simulink model "Optical_Movement_Detection"  (Simulink 7.5)
settings: Solver=ode45  StartTime=0.0  StopTime=inf  RelTol=1e-3
values from neighbouring files (symbols this model uses):
  D = 1    [Copter_Animation.m]
  HSE_Bottom_1 = imresize(imread('D:\GoogleMapsBilder\PAR\HSE_Bottom_1.jpg'), 1)    [TESTS_Optical_Flow_Scenarios.m]
undefined symbols (not defined in the file or in its folder): dfilt, fspecial, imresize, Kanade, Low, Lucas, Rec, SDTV
libraries: simulink x17, dspobslib x12, vipgeotforms x5, dspsigops x4, dspmtrx3 x3, vipanalysis x3, dspstat3 x3, vipconversions x2, dspswit3 x2, vipsrcs x2, dsparch4 x1, dspsrcs4 x1
(part 2 of 2)

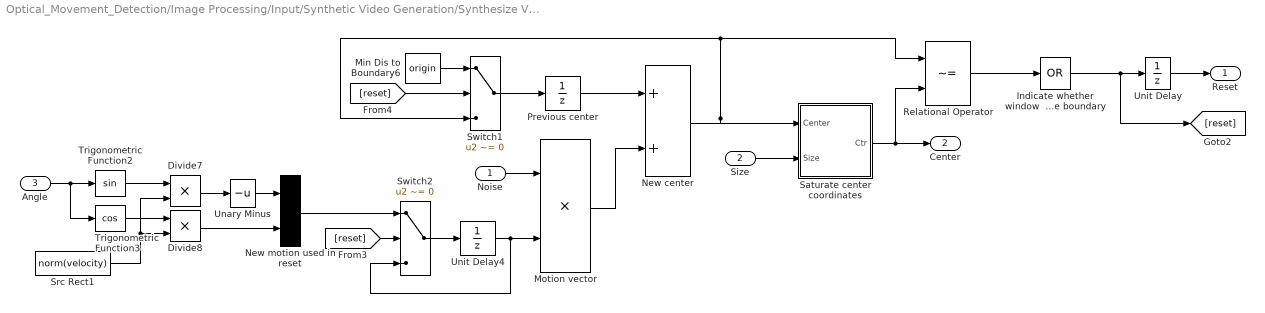
== system Optical_Movement_Detection/Image Processing/Input/Synthetic Video Generation/Synthesize Video/Center Locations ==
  Noise : Inport
  Size : Inport  Port=2  OutDataType=sfix(16)  OutScaling=2^0
  Angle : Inport  Port=3
  Divide7 : Product  Inputs=**  OutDataType=sfix(16)  OutScaling=2^-10
  Divide8 : Product  Inputs=**  OutDataType=sfix(16)  OutScaling=2^-10
  Indicate whether window  hit image boundary : Logic  Operator=OR  Inputs=1  AllPortsSameDT=off  OutDataTypeMode=boolean  OutDataTypeStr=boolean
  Min Dis to Boundary6 : Constant  Value=origin  OutDataType=sfix(16)  OutScaling=2^0
  Motion vector : Product  Inputs=**  OutDataType=sfix(16)  OutScaling=2^-10
  New center : Sum  OutDataType=sfix(16)  OutScaling=2^-10
  New motion used in reset : Concatenate  Mode=Vector
  Previous center : UnitDelay  X0=origin  SampleTime=-1
  Relational Operator : RelationalOperator  Operator=~=  LogicOutDataTypeMode=boolean  OutDataTypeStr=boolean
  Saturate center coordinates : Subsystem
  Src Rect1 : Constant  Value=norm(velocity)  VectorParams1D=off  OutDataType=sfix(16)  OutScaling=2^0  OutDataTypeStr=Inherit: Inherit via back propagation
  Switch1 : Switch  Criteria=u2 ~= 0  OutDataType=sfix(16)  OutScaling=2^0
  Switch2 : Switch  Criteria=u2 ~= 0  OutDataType=sfix(16)  OutScaling=2^0
  Trigonometric Function2 : Trigonometry
  Trigonometric Function3 : Trigonometry  Operator=cos
  Unary Minus : UnaryMinus
  Unit Delay : UnitDelay  X0=1  SampleTime=-1
  Unit Delay4 : UnitDelay  X0=velocity  SampleTime=-1
  Reset : Outport
  Center : Outport  Port=2
  wires:
  Unit Delay4/1 -> Switch2/3, Motion vector/2
  Previous center/1 -> New center/1
  [reset] -> Switch1/2
  [reset] -> Switch2/2
  Divide7/1 -> Unary Minus/1
  Unary Minus/1 -> New motion used in reset/1
  Divide8/1 -> New motion used in reset/2
  Src Rect1/1 -> Divide8/2, Divide7/2
  Switch1/1 -> Previous center/1
  Min Dis to Boundary6/1 -> Switch1/1
  Switch2/1 -> Unit Delay4/1
  New motion used in reset/1 -> Switch2/1
  Trigonometric Function3/1 -> Divide8/1
  Trigonometric Function2/1 -> Divide7/1
  Angle/1 -> Trigonometric Function3/1, Trigonometric Function2/1
  Relational Operator/1 -> Indicate whether window  hit image boundary/1
  Indicate whether window  hit image boundary/1 -> [reset], Unit Delay/1
  Saturate center coordinates/1(Ctr) -> Center/1, Relational Operator/2
  Size/1 -> Saturate center coordinates/2(Size)
  New center/1 -> Switch1/3, Relational Operator/1, Saturate center coordinates/1(Center)
  Unit Delay/1 -> Reset/1
  Motion vector/1 -> New center/2
  Noise/1 -> Motion vector/1

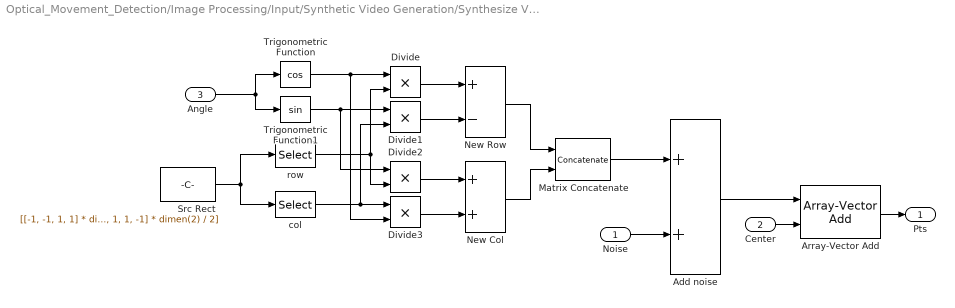
== system Optical_Movement_Detection/Image Processing/Input/Synthetic Video Generation/Synthesize Video/Corner Locations ==
  Noise : Inport
  Center : Inport  Port=2
  Angle : Inport  Port=3
  Add noise : Sum  OutDataType=sfix(16)  OutScaling=2^-10
  Array-Vector Add : dspmtrx3/Array-Vector Add  DialogController=dspDDGCreate  DialogControllerArgs=DataTag6  Dimension=1  V_Source=Input port  V_VectFromMask=[0.5 0.25]  firstCoeffDataTypeStr=Inherit: Same word length as input  firstCoeffLastDataTypeStr=Inherit: Same word length as input  firstCoeffMin=[]  firstCoeffMax=[]  outputDataTypeStr=Inherit: Same as accumulator  outputLastDataTypeStr=Inherit: Same as accumulator  outputMin=[]  outputMax=[]  roundingMode=Floor  overflowMode=off
  Divide{,1..3} (4 alike) : Product  Inputs=**  OutDataType=sfix(16)  OutScaling=2^-10
  Matrix Concatenate : Concatenate  Mode=Multidimensional array
  New Col : Sum  OutDataType=sfix(16)  OutScaling=2^-10
  New Row : Sum  Inputs=+-  OutDataType=sfix(16)  OutScaling=2^-10
  Src Rect : Constant  Value=[[-1, -1, 1, 1] * dimen(1) / 2; [-1, 1, 1, -1] * dimen(2) / 2]  OutDataType=sfix(16)  OutScaling=2^0
  Trigonometric Function : Trigonometry  Operator=cos
  Trigonometric Function1 : Trigonometry
  col : Selector  NumberOfDimensions=2  IndexMode=Zero-based  InputPortWidth=3  IndexOptions=Index vector (dialog),Select all  Indices=1,1  OutputSizes=1,1
  row : Selector  NumberOfDimensions=2  IndexMode=Zero-based  InputPortWidth=3  IndexOptions=Index vector (dialog),Select all  Indices=0,1  OutputSizes=1,1
  Pts : Outport
  wires:
  Noise/1 -> Add noise/2
  Center/1 -> Array-Vector Add/2
  Array-Vector Add/1 -> Pts/1
  Src Rect/1 -> col/1, row/1
  Divide2/1 -> New Col/1
  Divide3/1 -> New Col/2
  New Row/1 -> Matrix Concatenate/1
  New Col/1 -> Matrix Concatenate/2
  Matrix Concatenate/1 -> Add noise/1
  Angle/1 -> Trigonometric Function/1, Trigonometric Function1/1
  Divide/1 -> New Row/1
  Divide1/1 -> New Row/2
  Trigonometric Function/1 -> Divide3/2, Divide/1
  Trigonometric Function1/1 -> Divide2/1, Divide1/1
  row/1 -> Divide2/2, Divide/2
  col/1 -> Divide1/2, Divide3/1
  Add noise/1 -> Array-Vector Add/1

== system Optical_Movement_Detection/Image Processing/Optical Flow/Corner Features OF/Corner Matching/Calculate Distances ==
  F1 : Inport  OutDataType=sfix(16)  OutScaling=2^0
  N1 : Inport  Port=2  OutDataType=sfix(16)  OutScaling=2^0
  F2 : Inport  Port=3  OutDataType=sfix(16)  OutScaling=2^0
  N2 : Inport  Port=4  OutDataType=sfix(16)  OutScaling=2^0
  For Iterator Subsystem : Subsystem  TreatAsAtomicUnit=on
  Initial Values1 : Constant  Value=maxNum  OutDataType=sfix(16)  OutScaling=2^0  OutDataTypeStr=Inherit: Inherit via back propagation  SampleTime=-1
  Initial Values2 : Constant  Value=maxNum  OutDataType=sfix(16)  OutScaling=2^0  OutDataTypeStr=Inherit: Inherit via back propagation  SampleTime=-1
  MinMax1 : MinMax  Inputs=2  OutDataType=sfix(16)  OutScaling=2^0
  MinMax2 : MinMax  Inputs=2  OutDataType=sfix(16)  OutScaling=2^0
  Dis : Outport  OutDataType=sfix(16)  OutScaling=2^0
  wires:
  MinMax2/1 -> For Iterator Subsystem/4(N2)
  F2/1 -> For Iterator Subsystem/3(F2)
  MinMax1/1 -> For Iterator Subsystem/2(N1)
  F1/1 -> For Iterator Subsystem/1(F1)
  For Iterator Subsystem/1(Dis) -> Dis/1
  N2/1 -> MinMax2/2
  Initial Values2/1 -> MinMax2/1
  N1/1 -> MinMax1/2
  Initial Values1/1 -> MinMax1/1

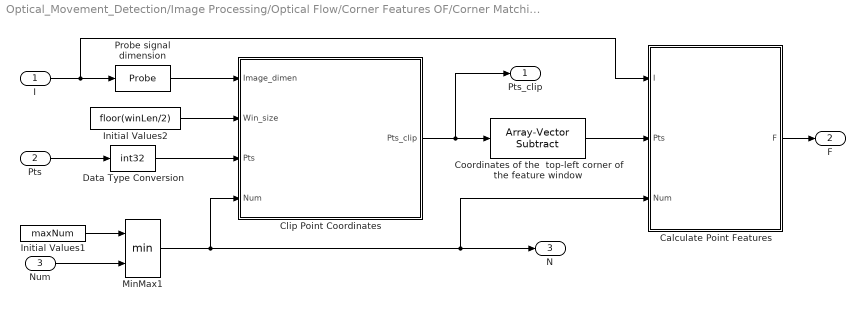
== system Optical_Movement_Detection/Image Processing/Optical Flow/Corner Features OF/Corner Matching/Calculate Features ==
  I : Inport  OutDataType=sfix(16)  OutScaling=2^0
  Pts : Inport  Port=2  OutDataType=sfix(16)  OutScaling=2^0
  Num : Inport  Port=3  OutDataType=sfix(16)  OutScaling=2^0
  Calculate Point Features : Subsystem
  Clip Point Coordinates : Subsystem
  Coordinates of the  top-left corner of the feature window : dspmtrx3/Array-Vector Subtract  DialogController=dspDDGCreate  DialogControllerArgs=DataTag10  Dimension=1  V_Source=Dialog parameter  V_VectFromMask=floor([winLen; winLen] / 2)  firstCoeffDataTypeStr=Inherit: Same word length as input  firstCoeffLastDataTypeStr=Inherit: Same word length as input  firstCoeffMin=[]  firstCoeffMax=[]  outputMin=[]  outputMax=[]  roundingMode=Floor  overflowMode=off
  Data Type Conversion : DataTypeConversion  OutDataTypeMode=int32  OutDataType=sfix(16)  OutScaling=2^0  OutDataTypeStr=int32
  Initial Values1 : Constant  Value=maxNum  OutDataType=sfix(16)  OutScaling=2^0  OutDataTypeStr=Inherit: Inherit via back propagation  SampleTime=-1
  Initial Values2 : Constant  Value=floor(winLen/2)  OutDataType=sfix(16)  OutScaling=2^0  OutDataTypeStr=Inherit: Inherit via back propagation  SampleTime=-1
  MinMax1 : MinMax  Inputs=2  OutDataType=sfix(16)  OutScaling=2^0
  Probe signal dimension : Probe  ProbeWidth=off  ProbeSampleTime=off  ProbeComplexSignal=off  ProbeSignalDimensions=on  ProbeDimensionsDataType=int32
  Pts_clip : Outport  OutDataType=sfix(16)  OutScaling=2^0
  F : Outport  Port=2  OutDataType=sfix(16)  OutScaling=2^0
  N : Outport  Port=3  OutDataType=sfix(16)  OutScaling=2^0
  wires:
  Data Type Conversion/1 -> Clip Point Coordinates/3(Pts)
  MinMax1/1 -> N/1, Calculate Point Features/3(Num), Clip Point Coordinates/4(Num)
  Coordinates of the  top-left corner of the feature window/1 -> Calculate Point Features/2(Pts)
  Clip Point Coordinates/1(Pts_clip) -> Coordinates of the  top-left corner of the feature window/1, Pts_clip/1
  Pts/1 -> Data Type Conversion/1
  Initial Values2/1 -> Clip Point Coordinates/2(Win_size)
  Probe signal dimension/1 -> Clip Point Coordinates/1(Image_dimen)
  I/1 -> Calculate Point Features/1(I), Probe signal dimension/1
  Initial Values1/1 -> MinMax1/1
  Num/1 -> MinMax1/2
  Calculate Point Features/1(F) -> F/1

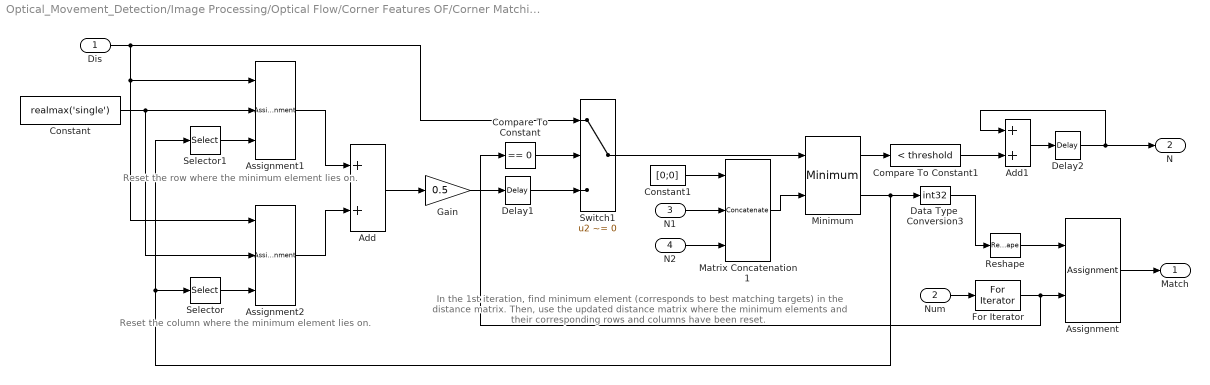
== system Optical_Movement_Detection/Image Processing/Optical Flow/Corner Features OF/Corner Matching/Find Best Matches ==
  note: In the 1st iteration, find minimum element (corresponds to
      | best matching targets) in the distance matrix. Then, use the
      | updated distance matrix where the minimum elements and
      | their  corresponding rows and columns have been reset.
  note: Reset the column where the
      | minimum element lies on.
  note: Reset the row where the
      | minimum element lies on.
  Dis : Inport  OutDataType=sfix(16)  OutScaling=2^0
  Num : Inport  Port=2  OutDataType=sfix(16)  OutScaling=2^0
  N1 : Inport  Port=3  OutDataType=sfix(16)  OutScaling=2^0
  N2 : Inport  Port=4  OutDataType=sfix(16)  OutScaling=2^0
  Add : Sum  OutDataType=sfix(16)  OutScaling=2^-10
  Add1 : Sum  OutDataTypeMode=int32  OutDataType=sfix(16)  OutScaling=2^-10  OutDataTypeStr=int32
  Assignment : Assignment  NumberOfDimensions=2  IndexMode=Zero-based  OutputInitialize=Specify size for each dimension in table  IndexOptions=Assign all,Index vector (port)  Indices=-1,-1  OutputSizes=2,maxNum
  Assignment1 : Assignment  NumberOfDimensions=2  IndexMode=Zero-based  IndexOptions=Index vector (port),Assign all  Indices=1,-1  OutputSizes=1,1
  Assignment2 : Assignment  NumberOfDimensions=2  IndexMode=Zero-based  IndexOptions=Assign all,Index vector (port)  Indices=-1,-1  OutputSizes=1,1
  Compare To Constant : simulink/Logic and Bit Operations/Compare To Constant  SystemSampleTime=-1  relop===  const=0  LogicOutDataTypeMode=boolean  ZeroCross=off
  Compare To Constant1 : simulink/Logic and Bit Operations/Compare To Constant  SystemSampleTime=-1  relop=<  const=threshold  LogicOutDataTypeMode=uint8  ZeroCross=off
  Constant : Constant  Value=realmax('single')  VectorParams1D=off  OutDataType=sfix(16)  OutScaling=2^0  OutDataTypeStr=Inherit: Inherit via back propagation
  Constant1 : Constant  Value=[0;0]  VectorParams1D=off  OutDataType=sfix(16)  OutScaling=2^0  OutDataTypeStr=Inherit: Inherit via back propagation
  Data Type  Conversion3 : DataTypeConversion  OutDataTypeMode=int32  OutDataType=sfix(16)  OutScaling=2^0  OutDataTypeStr=int32  SaturateOnIntegerOverflow=on  RndMeth=Zero
  Delay1 : dspsigops/Delay  dly_unit=Samples  delay=1  ic_detail=off  dif_ic_for_ch=off  dif_ic_for_dly=off  ic=0  reset_popup=None
  Delay2 : dspsigops/Delay  dly_unit=Samples  delay=1  ic_detail=off  dif_ic_for_ch=off  dif_ic_for_dly=off  ic=0  reset_popup=None
  For Iterator : ForIterator  ResetStates=reset  IterationSource=external  IterationLimit=expLaneNum  IndexMode=Zero-based
  Gain : Gain  Gain=0.5  ParameterDataType=sfix(16)  ParameterScaling=2^0  OutDataType=sfix(16)  OutScaling=2^0
  Matrix Concatenation1 : Concatenate  NumInputs=3  Mode=Multidimensional array
  Minimum : dspstat3/Minimum  DialogController=dspDDGCreate  DialogControllerArgs=DataTag11  fcn=Value and Index  reset=None  indexBase=Zero  operateOver=Entire input  Dimension=1  colComp=on  operation=minimum  roiEnable=on  roiType=Rectangles  roiPortion=Entire ROI  roiOutput=Individual statistics for each ROI  roiFlag=off  roundingMode=Floor  overflowMode=off
  Reshape : Reshape  OutputDimensionality=Column vector (2-D)
  Selector : Selector  IndexMode=Zero-based  InputPortWidth=2  IndexOptions=Index vector (dialog)  Indices=1  OutputSizes=1
  Selector1 : Selector  IndexMode=Zero-based  InputPortWidth=2  IndexOptions=Index vector (dialog)  Indices=0  OutputSizes=1
  Switch1 : Switch  Criteria=u2 ~= 0  OutDataType=sfix(16)  OutScaling=2^0
  Match : Outport  OutDataType=sfix(16)  OutScaling=2^0
  N : Outport  Port=2  OutDataType=sfix(16)  OutScaling=2^0
  wires:
  Gain/1 -> Delay1/1
  Minimum/1 -> Compare To Constant1/1
  Compare To Constant1/1 -> Add1/2
  Delay2/1 -> Add1/1, N/1
  Add1/1 -> Delay2/1
  Num/1 -> For Iterator/1
  Data Type  Conversion3/1 -> Reshape/1
  Compare To Constant/1 -> Switch1/2
  For Iterator/1 -> Compare To Constant/1, Assignment/2
  Switch1/1 -> Minimum/1
  Dis/1 -> Switch1/1, Assignment2/1, Assignment1/1
  Delay1/1 -> Switch1/3
  Assignment/1 -> Match/1
  Selector1/1 -> Assignment1/3
  Assignment1/1 -> Add/1
  Assignment2/1 -> Add/2
  Add/1 -> Gain/1
  Minimum/2 -> Data Type  Conversion3/1, Selector/1, Selector1/1
  Constant/1 -> Assignment1/2, Assignment2/2
  Selector/1 -> Assignment2/3
  Constant1/1 -> Matrix Concatenation1/1
  N1/1 -> Matrix Concatenation1/2
  N2/1 -> Matrix Concatenation1/3
  Matrix Concatenation1/1 -> Minimum/2
  Reshape/1 -> Assignment/1

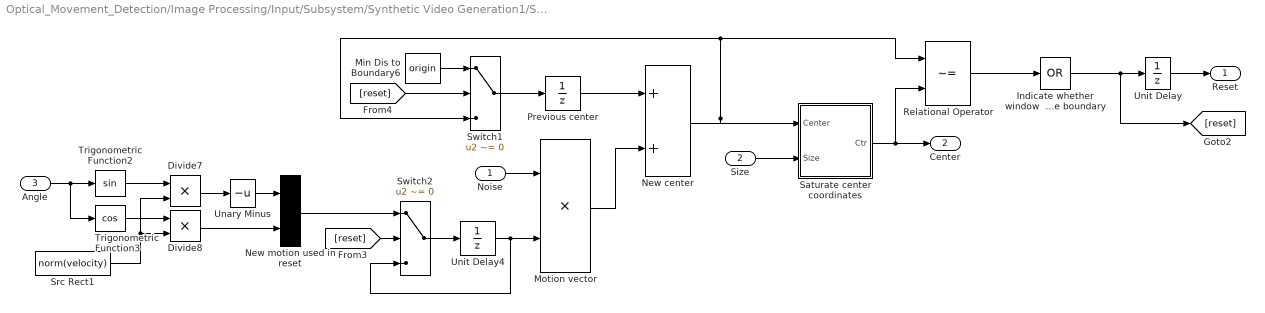
== system Optical_Movement_Detection/Image Processing/Input/Subsystem/Synthetic Video Generation1/Synthesize Video/Center Locations ==
  Noise : Inport
  Size : Inport  Port=2  OutDataType=sfix(16)  OutScaling=2^0
  Angle : Inport  Port=3
  Divide7 : Product  Inputs=**  OutDataType=sfix(16)  OutScaling=2^-10
  Divide8 : Product  Inputs=**  OutDataType=sfix(16)  OutScaling=2^-10
  Indicate whether window  hit image boundary : Logic  Operator=OR  Inputs=1  AllPortsSameDT=off  OutDataTypeMode=boolean  OutDataTypeStr=boolean
  Min Dis to Boundary6 : Constant  Value=origin  OutDataType=sfix(16)  OutScaling=2^0
  Motion vector : Product  Inputs=**  OutDataType=sfix(16)  OutScaling=2^-10
  New center : Sum  OutDataType=sfix(16)  OutScaling=2^-10
  New motion used in reset : Concatenate  Mode=Vector
  Previous center : UnitDelay  X0=origin  SampleTime=-1
  Relational Operator : RelationalOperator  Operator=~=  LogicOutDataTypeMode=boolean  OutDataTypeStr=boolean
  Saturate center coordinates : Subsystem
  Src Rect1 : Constant  Value=norm(velocity)  VectorParams1D=off  OutDataType=sfix(16)  OutScaling=2^0  OutDataTypeStr=Inherit: Inherit via back propagation
  Switch1 : Switch  Criteria=u2 ~= 0  OutDataType=sfix(16)  OutScaling=2^0
  Switch2 : Switch  Criteria=u2 ~= 0  OutDataType=sfix(16)  OutScaling=2^0
  Trigonometric Function2 : Trigonometry
  Trigonometric Function3 : Trigonometry  Operator=cos
  Unary Minus : UnaryMinus
  Unit Delay : UnitDelay  X0=1  SampleTime=-1
  Unit Delay4 : UnitDelay  X0=velocity  SampleTime=-1
  Reset : Outport
  Center : Outport  Port=2
  wires:
  Unit Delay4/1 -> Switch2/3, Motion vector/2
  Previous center/1 -> New center/1
  [reset] -> Switch1/2
  [reset] -> Switch2/2
  Divide7/1 -> Unary Minus/1
  Unary Minus/1 -> New motion used in reset/1
  Divide8/1 -> New motion used in reset/2
  Src Rect1/1 -> Divide8/2, Divide7/2
  Switch1/1 -> Previous center/1
  Min Dis to Boundary6/1 -> Switch1/1
  Switch2/1 -> Unit Delay4/1
  New motion used in reset/1 -> Switch2/1
  Trigonometric Function3/1 -> Divide8/1
  Trigonometric Function2/1 -> Divide7/1
  Angle/1 -> Trigonometric Function3/1, Trigonometric Function2/1
  Relational Operator/1 -> Indicate whether window  hit image boundary/1
  Indicate whether window  hit image boundary/1 -> [reset], Unit Delay/1
  Saturate center coordinates/1(Ctr) -> Center/1, Relational Operator/2
  Size/1 -> Saturate center coordinates/2(Size)
  New center/1 -> Switch1/3, Relational Operator/1, Saturate center coordinates/1(Center)
  Unit Delay/1 -> Reset/1
  Motion vector/1 -> New center/2
  Noise/1 -> Motion vector/1

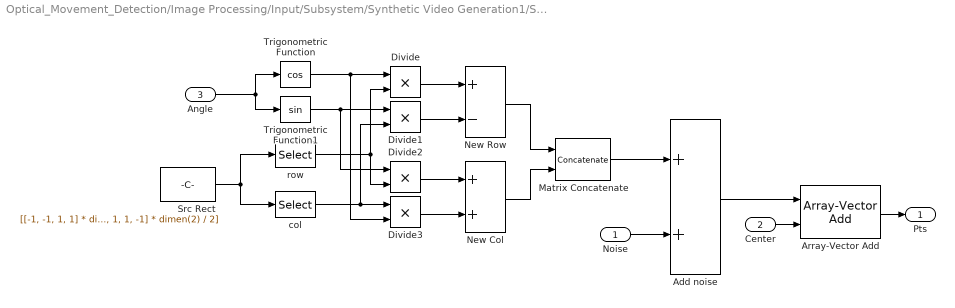
== system Optical_Movement_Detection/Image Processing/Input/Subsystem/Synthetic Video Generation1/Synthesize Video/Corner Locations ==
  Noise : Inport
  Center : Inport  Port=2
  Angle : Inport  Port=3
  Add noise : Sum  OutDataType=sfix(16)  OutScaling=2^-10
  Array-Vector Add : dspmtrx3/Array-Vector Add  DialogController=dspDDGCreate  DialogControllerArgs=DataTag2  Dimension=1  V_Source=Input port  V_VectFromMask=[0.5 0.25]  firstCoeffDataTypeStr=Inherit: Same word length as input  firstCoeffLastDataTypeStr=Inherit: Same word length as input  firstCoeffMin=[]  firstCoeffMax=[]  outputDataTypeStr=Inherit: Same as accumulator  outputLastDataTypeStr=Inherit: Same as accumulator  outputMin=[]  outputMax=[]  roundingMode=Floor  overflowMode=off
  Divide{,1..3} (4 alike) : Product  Inputs=**  OutDataType=sfix(16)  OutScaling=2^-10
  Matrix Concatenate : Concatenate  Mode=Multidimensional array
  New Col : Sum  OutDataType=sfix(16)  OutScaling=2^-10
  New Row : Sum  Inputs=+-  OutDataType=sfix(16)  OutScaling=2^-10
  Src Rect : Constant  Value=[[-1, -1, 1, 1] * dimen(1) / 2; [-1, 1, 1, -1] * dimen(2) / 2]  OutDataType=sfix(16)  OutScaling=2^0
  Trigonometric Function : Trigonometry  Operator=cos
  Trigonometric Function1 : Trigonometry
  col : Selector  NumberOfDimensions=2  IndexMode=Zero-based  InputPortWidth=3  IndexOptions=Index vector (dialog),Select all  Indices=1,1  OutputSizes=1,1
  row : Selector  NumberOfDimensions=2  IndexMode=Zero-based  InputPortWidth=3  IndexOptions=Index vector (dialog),Select all  Indices=0,1  OutputSizes=1,1
  Pts : Outport
  wires:
  Noise/1 -> Add noise/2
  Center/1 -> Array-Vector Add/2
  Array-Vector Add/1 -> Pts/1
  Src Rect/1 -> col/1, row/1
  Divide2/1 -> New Col/1
  Divide3/1 -> New Col/2
  New Row/1 -> Matrix Concatenate/1
  New Col/1 -> Matrix Concatenate/2
  Matrix Concatenate/1 -> Add noise/1
  Angle/1 -> Trigonometric Function/1, Trigonometric Function1/1
  Divide/1 -> New Row/1
  Divide1/1 -> New Row/2
  Trigonometric Function/1 -> Divide3/2, Divide/1
  Trigonometric Function1/1 -> Divide2/1, Divide1/1
  row/1 -> Divide2/2, Divide/2
  col/1 -> Divide1/2, Divide3/1
  Add noise/1 -> Array-Vector Add/1

== system Optical_Movement_Detection/Image Processing/Input/Synthetic Video Generation/Synthesize Video/Center Locations/Saturate center coordinates ==
  Center : Inport
  Size : Inport  Port=2
  Center2 : Sum  Inputs=-+  OutDataType=sfix(16)  OutScaling=2^-10
  Min Dis to Boundary : Constant  Value=kron([ceil(sqrt(dimen(1)^2+dimen(2)^2)/2)], [1; 1])  OutDataType=sfix(16)  OutScaling=2^0
  MinMax : MinMax  Function=max  Inputs=2  OutDataType=sfix(16)  OutScaling=2^0
  MinMax1 : MinMax  Inputs=2  OutDataType=sfix(16)  OutScaling=2^0
  row1 : Selector  IndexMode=Zero-based  InputPortWidth=3  IndexOptions=Index vector (dialog)  Indices=[0 1]  OutputSizes=1
  Ctr : Outport
  wires:
  Size/1 -> row1/1
  MinMax1/1 -> Ctr/1
  Center/1 -> MinMax/1
  Center2/1 -> MinMax1/2
  MinMax/1 -> MinMax1/1
  row1/1 -> Center2/2
  Min Dis to Boundary/1 -> Center2/1, MinMax/2

== system Optical_Movement_Detection/Image Processing/Optical Flow/Corner Features OF/Corner Matching/Calculate Distances/For Iterator Subsystem ==
  F1 : Inport  OutDataType=sfix(16)  OutScaling=2^0
  N1 : Inport  Port=2  OutDataType=sfix(16)  OutScaling=2^0
  F2 : Inport  Port=3  OutDataType=sfix(16)  OutScaling=2^0
  N2 : Inport  Port=4  OutDataType=sfix(16)  OutScaling=2^0
  For Iterator : ForIterator  IterationSource=external  IndexMode=Zero-based
  For Iterator Subsystem : Subsystem  TreatAsAtomicUnit=on
  Select feature  for 1 corner : Selector  NumberOfDimensions=2  IndexMode=Zero-based  InputPortWidth=2  IndexOptions=Select all,Index vector (port)  Indices=0,1  OutputSizes=1,1
  Update feature  for a corner : Assignment  NumberOfDimensions=2  IndexMode=Zero-based  OutputInitialize=Specify size for each dimension in table  IndexOptions=Assign all,Index vector (port)  Indices=1,1  OutputSizes=maxNum,maxNum
  Dis : Outport  OutDataType=sfix(16)  OutScaling=2^0
  wires:
  Update feature  for a corner/1 -> Dis/1
  N1/1 -> For Iterator Subsystem/2(N1)
  F1/1 -> For Iterator Subsystem/1(F1)
  Select feature  for 1 corner/1 -> For Iterator Subsystem/3(f2)
  F2/1 -> Select feature  for 1 corner/1
  For Iterator/1 -> Select feature  for 1 corner/2, Update feature  for a corner/2
  N2/1 -> For Iterator/1
  For Iterator Subsystem/1(Dis) -> Update feature  for a corner/1

== system Optical_Movement_Detection/Image Processing/Optical Flow/Corner Features OF/Corner Matching/Calculate Features/Calculate Point Features ==
  note: Calculate feature for a corner.
  I : Inport
  Pts : Inport  Port=2
  Num : Inport  Port=3
  For Iterator : ForIterator  IterationSource=external  IndexMode=Zero-based
  Reshape : Reshape  OutputDimensionality=Column vector (2-D)
  Selector : Selector  NumberOfDimensions=2  IndexMode=Zero-based  InputPortWidth=3  IndexOptions=Starting index (port),Starting index (port)  Indices=[1 3],1  OutputSizes=winLen,winLen
  Selector1 : Selector  NumberOfDimensions=2  IndexMode=Zero-based  InputPortWidth=3  IndexOptions=Select all,Index vector (port)  Indices=[1 3],1  OutputSizes=9,9
  Selector2 : Selector  IndexMode=Zero-based  InputPortWidth=2  IndexOptions=Index vector (dialog)  Indices=0  OutputSizes=9
  Selector3 : Selector  IndexMode=Zero-based  InputPortWidth=2  IndexOptions=Index vector (dialog)  Indices=1  OutputSizes=9
  Update Feature  for a Corner : Assignment  NumberOfDimensions=2  IndexMode=Zero-based  OutputInitialize=Specify size for each dimension in table  IndexOptions=Assign all,Index vector (port)  Indices=1,1  OutputSizes=winLen^2,maxNum
  F : Outport
  wires:
  Selector3/1 -> Selector/3
  Selector2/1 -> Selector/2
  Num/1 -> For Iterator/1
  Update Feature  for a Corner/1 -> F/1
  Pts/1 -> Selector1/1
  I/1 -> Selector/1
  Reshape/1 -> Update Feature  for a Corner/1
  Selector/1 -> Reshape/1
  Selector1/1 -> Selector2/1, Selector3/1
  For Iterator/1 -> Update Feature  for a Corner/2, Selector1/2

== system Optical_Movement_Detection/Image Processing/Optical Flow/Corner Features OF/Corner Matching/Calculate Features/Clip Point Coordinates ==
  Image_dimen : Inport  OutDataType=sfix(16)  OutScaling=2^0
  Win_size : Inport  Port=2  OutDataType=sfix(16)  OutScaling=2^0
  Pts : Inport  Port=3
  Num : Inport  Port=4
  Add : Sum  Inputs=-+  OutDataType=sfix(16)  OutScaling=2^-10
  Bias : Bias  Bias=-1
  Clip row/col coordinates : Subsystem
  For i = 0: 1 (select row/col) : ForIterator  IterationLimit=2  IndexMode=Zero-based
  Selector1 : Selector  NumberOfDimensions=2  IndexMode=Zero-based  InputPortWidth=3  IndexOptions=Index vector (port),Select all  Indices=[1 3],1  OutputSizes=9,9
  Selector2 : Selector  IndexMode=Zero-based  InputPortWidth=2  IndexOptions=Index vector (port)  Indices=[1 3]  OutputSizes=9
  Update Coordinates : Assignment  NumberOfDimensions=2  IndexMode=Zero-based  IndexOptions=Index vector (port),Assign all  Indices=1,1  OutputSizes=81,50
  Pts_clip : Outport  OutDataType=sfix(16)  OutScaling=2^0
  wires:
  Selector2/1 -> Add/2
  For i = 0: 1 (select row/col)/1 -> Selector1/2, Selector2/2, Update Coordinates/3
  Clip row/col coordinates/1(Coordinates_clip) -> Update Coordinates/2
  Bias/1 -> Clip row/col coordinates/2(High)
  Update Coordinates/1 -> Pts_clip/1
  Num/1 -> Clip row/col coordinates/4(Num)
  Selector1/1 -> Clip row/col coordinates/3(Coordinates)
  Win_size/1 -> Add/1, Clip row/col coordinates/1(Low)
  Add/1 -> Bias/1
  Image_dimen/1 -> Selector2/1
  Pts/1 -> Update Coordinates/1, Selector1/1

== system Optical_Movement_Detection/Image Processing/Input/Subsystem/Synthetic Video Generation1/Synthesize Video/Center Locations/Saturate center coordinates ==
  Center : Inport
  Size : Inport  Port=2
  Center2 : Sum  Inputs=-+  OutDataType=sfix(16)  OutScaling=2^-10
  Min Dis to Boundary : Constant  Value=kron([ceil(sqrt(dimen(1)^2+dimen(2)^2)/2)], [1; 1])  OutDataType=sfix(16)  OutScaling=2^0
  MinMax : MinMax  Function=max  Inputs=2  OutDataType=sfix(16)  OutScaling=2^0
  MinMax1 : MinMax  Inputs=2  OutDataType=sfix(16)  OutScaling=2^0
  row1 : Selector  IndexMode=Zero-based  InputPortWidth=3  IndexOptions=Index vector (dialog)  Indices=[0 1]  OutputSizes=1
  Ctr : Outport
  wires:
  Size/1 -> row1/1
  MinMax1/1 -> Ctr/1
  Center/1 -> MinMax/1
  Center2/1 -> MinMax1/2
  MinMax/1 -> MinMax1/1
  row1/1 -> Center2/2
  Min Dis to Boundary/1 -> Center2/1, MinMax/2

== system Optical_Movement_Detection/Image Processing/Optical Flow/Corner Features OF/Corner Matching/Calculate Distances/For Iterator Subsystem/For Iterator Subsystem ==
  F1 : Inport  OutDataType=sfix(16)  OutScaling=2^0
  N1 : Inport  Port=2  OutDataType=sfix(16)  OutScaling=2^0
  f2 : Inport  Port=3  OutDataType=sfix(16)  OutScaling=2^0
  Distance between two feature vectors : Subsystem
  For Iterator : ForIterator  IterationSource=external  IndexMode=Zero-based
  Select feature  for 1 corner : Selector  NumberOfDimensions=2  IndexMode=Zero-based  InputPortWidth=2  IndexOptions=Select all,Index vector (port)  Indices=0,1  OutputSizes=1,1
  Update feature  for a corner : Assignment  NumberOfDimensions=2  IndexMode=Zero-based  OutputInitialize=Specify size for each dimension in table  IndexOptions=Index vector (port),Assign all  Indices=1,1  OutputSizes=maxNum,1
  Dis : Outport  OutDataType=sfix(16)  OutScaling=2^0
  wires:
  Select feature  for 1 corner/1 -> Distance between two feature vectors/1(f1)
  f2/1 -> Distance between two feature vectors/2(f2)
  Update feature  for a corner/1 -> Dis/1
  F1/1 -> Select feature  for 1 corner/1
  For Iterator/1 -> Select feature  for 1 corner/2, Update feature  for a corner/2
  N1/1 -> For Iterator/1
  Distance between two feature vectors/1(dis) -> Update feature  for a corner/1

== system Optical_Movement_Detection/Image Processing/Optical Flow/Corner Features OF/Corner Matching/Calculate Features/Clip Point Coordinates/Clip row/col coordinates ==
  Low : Inport  OutDataType=sfix(16)  OutScaling=2^0
  High : Inport  Port=2  OutDataType=sfix(16)  OutScaling=2^0
  Coordinates : Inport  Port=3
  Num : Inport  Port=4  OutDataType=sfix(16)  OutScaling=2^0
  Clip a Coordinate : Subsystem
  For Iterator : ForIterator  IterationSource=external  IterationLimit=2  IndexMode=Zero-based
  Select Coordinate of a Point : Selector  NumberOfDimensions=2  IndexMode=Zero-based  InputPortWidth=3  IndexOptions=Select all,Index vector (port)  Indices=[1 3],1  OutputSizes=9,1
  Update Feature  for a Corner : Assignment  NumberOfDimensions=2  IndexMode=Zero-based  IndexOptions=Assign all,Index vector (port)  Indices=1,1  OutputSizes=81,50
  Coordinates_clip : Outport  OutDataType=sfix(16)  OutScaling=2^0
  wires:
  Clip a Coordinate/1(Coordinate_clip) -> Update Feature  for a Corner/2
  Update Feature  for a Corner/1 -> Coordinates_clip/1
  High/1 -> Clip a Coordinate/2(High)
  Low/1 -> Clip a Coordinate/1(Low)
  Select Coordinate of a Point/1 -> Clip a Coordinate/3(Coordinate)
  Num/1 -> For Iterator/1
  Coordinates/1 -> Update Feature  for a Corner/1, Select Coordinate of a Point/1
  For Iterator/1 -> Select Coordinate of a Point/2, Update Feature  for a Corner/3

== system Optical_Movement_Detection/Image Processing/Optical Flow/Corner Features OF/Corner Matching/Calculate Distances/For Iterator Subsystem/For Iterator Subsystem/Distance between two feature vectors ==
  f1 : Inport  OutDataType=sfix(16)  OutScaling=2^0
  f2 : Inport  Port=2  OutDataType=sfix(16)  OutScaling=2^0
  Abs : Abs  OutDataType=sfix(16)  OutScaling=2^0
  Add : Sum  Inputs=+-  OutDataType=sfix(16)  OutScaling=2^-10
  Sum of Elements : Sum  Inputs=+  OutDataType=sfix(16)  OutScaling=2^-10
  dis : Outport  OutDataType=sfix(16)  OutScaling=2^0
  wires:
  Sum of Elements/1 -> dis/1
  Abs/1 -> Sum of Elements/1
  Add/1 -> Abs/1
  f2/1 -> Add/2
  f1/1 -> Add/1

== system Optical_Movement_Detection/Image Processing/Optical Flow/Corner Features OF/Corner Matching/Calculate Features/Clip Point Coordinates/Clip row/col coordinates/Clip a Coordinate ==
  Low : Inport  OutDataType=sfix(16)  OutScaling=2^0
  High : Inport  Port=2  OutDataType=sfix(16)  OutScaling=2^0
  Coordinate : Inport  Port=3  OutDataType=sfix(16)  OutScaling=2^0
  MinMax1 : MinMax  Function=max  Inputs=2  OutDataType=sfix(16)  OutScaling=2^0
  MinMax2 : MinMax  Inputs=2  OutDataType=sfix(16)  OutScaling=2^0
  Coordinate_clip : Outport  OutDataType=sfix(16)  OutScaling=2^0
  wires:
  MinMax2/1 -> Coordinate_clip/1
  High/1 -> MinMax2/2
  MinMax1/1 -> MinMax2/1
  Low/1 -> MinMax1/2
  Coordinate/1 -> MinMax1/1

== matlab function Image Processing/Optical Flow/Optical Flow Segmentation in Sectors Corner Features/Optical Flow Lines1 ==
  data: vel_Values input double; Cam_Img_Dim input double; vel_Lines output double; Omega_avg output double; scaleFactor parameter double size=1
function [vel_Lines, Omega_avg]=OpticalFlowLines(vel_Values, Cam_Img_Dim,scaleFactor) 

% Generates the coordinate points of optical flow lines

persistent first_time;
persistent X;
persistent Y;
persistent RV;
persistent CV;

%persistent Max_Vec_Length;

persistent Origin_Re;
persistent Origin_Im;

persistent Sec_1_Cnt;
persistent Sec_2_Cnt;
persistent Sec_3_Cnt;
persistent Sec_4_Cnt;

persistent Sec_1;
persistent Sec_2;
persistent Sec_3;
persistent Sec_4;

persistent R;
persistent C;
persistent Test_mat;
persistent med_vel_val;

%med_vel_val=median(vel_Values);
%[R C] = size(med_vel_val);
if isempty(first_time)
    first_time     = 1;
    Origin_Re = Cam_Img_Dim(1)/2%double(176);
    [R C] = size(vel_Values)
    Origin_Im = Cam_Img_Dim(2)/2%double(144);
end

Sec_1 = double(0);
Sec_2 = double(0);
Sec_3 = double(0);
Sec_4 = double(0);

Sec_1_Cnt = 1;
Sec_2_Cnt = 1;
Sec_3_Cnt = 1;
Sec_4_Cnt = 1;

%sectors
%       ^Im
%       |         
%   4   |  1
%-------------->Re
%   3   |  2
%       |

% for i=1:R
%     for k=1:C
%       j=vel_Values(i,k);
%     if(real(j)>=0) % Sec_1 or Sec_2
%         if(imag(j)>=0) %Sec_1
%             Sec_1_Cnt=Sec_1_Cnt+1;
%             Sec_1=Sec_1+double(abs(j))
%         else           %Sec_2
%             Sec_2_Cnt=Sec_2_Cnt+1;
%             Sec_2=Sec_2+double(abs(j))
%         end
%     else            % Sec_3 or Sec_4
%         if(imag(j)>=0) %Sec_4
%             Sec_4_Cnt=Sec_4_Cnt+1;
%             Sec_4=Sec_4+double(abs(j))
%         else           %Sec_3
%             Sec_3_Cnt=Sec_3_Cnt+1;
%             Sec_3=Sec_3+double(abs(j))
%         end
%     end
%     end
% end

%Other segm
for i=1:R
    for k=1:C
      j=vel_Values(i,k);
    if(real(j)>=0) % Sec_1 or Sec_2
        Sec_1_Cnt=Sec_1_Cnt+1;
        Sec_1=Sec_1+double(abs(real(j)));
        if(imag(j)>=0) %Sec_2
            Sec_2_Cnt=Sec_2_Cnt+1;
            Sec_2=Sec_2+double(imag(j));
        else           %Sec_4
            Sec_4_Cnt=Sec_4_Cnt+1;
            Sec_4=Sec_4+double(imag(j));
        end
    else            % Sec_3 or Sec_4
        Sec_3_Cnt=Sec_3_Cnt+1;
        Sec_3=Sec_3+double(abs(real(j)));
        if(imag(j)>=0) %Sec_2
            Sec_2_Cnt=Sec_2_Cnt+1;
            Sec_2=Sec_2+double(imag(j));
        else           %Sec_4
            Sec_4_Cnt=Sec_4_Cnt+1;
            Sec_4=Sec_4+double(imag(j));
        end
    end
    end
end


% Sec_1_Mat = vel_Values((real(vel_Values) >= 0) & (imag(vel_Values) >= 0));
% Sec_2_Mat = vel_Values((real(vel_Values) >= 0) & (imag(vel_Values) < 0));
% Sec_3_Mat = vel_Values((real(vel_Values) < 0) & (imag(vel_Values) < 0));
% Sec_4_Mat = vel_Values((real(vel_Values) < 0) & (imag(vel_Values) >= 0));


% Sec_1 = sum(abs(Sec_1_Mat)/(size(Sec_1_Mat, 1)*size(Sec_1_Mat, 2)));
% Sec_2 = sum(abs(Sec_1_Mat)/(size(Sec_1_Mat, 1)*size(Sec_1_Mat, 2)));
% Sec_3 = sum(abs(Sec_1_Mat)/(size(Sec_1_Mat, 1)*size(Sec_1_Mat, 2)));
% Sec_4 = sum(abs(Sec_1_Mat)/(size(Sec_1_Mat, 1)*size(Sec_1_Mat, 2)));

Sec_1 = Sec_1/Sec_1_Cnt;
Sec_2 = Sec_2/Sec_2_Cnt;
Sec_3 = Sec_3/Sec_3_Cnt;
Sec_4 = Sec_4/Sec_4_Cnt;

% Omega_Re_Plus = (scaleFactor*(Sec_1+Sec_2))/2
% Omega_Re_Minus = (scaleFactor*(Sec_3+Sec_4))/2
% Omega_Im_Plus = (scaleFactor*(Sec_1+Sec_4))/2
% Omega_Im_Minus = (scaleFactor*(Sec_3+Sec_2))/2

Omega_Re_Plus = scaleFactor*Sec_1; %Sec_2
Omega_Re_Minus = scaleFactor*Sec_3; %Sec_4
Omega_Im_Plus = scaleFactor*Sec_4; %Sec_1
Omega_Im_Minus = scaleFactor*Sec_2; %Sec_3

%Calculation of rotation

rotation_comp=min([abs(Omega_Re_Plus) abs(Omega_Re_Minus) abs(Omega_Im_Plus) abs(Omega_Im_Minus)]);

if(rotation_comp>0)
    Omega_avg = [abs(Omega_Re_Plus)-rotation_comp abs(Omega_Re_Minus)-rotation_comp abs(Omega_Im_Plus)-rotation_comp abs(Omega_Im_Minus)-rotation_comp rotation_comp];
else
    Omega_avg = [abs(Omega_Re_Plus) abs(Omega_Re_Minus) abs(Omega_Im_Plus) abs(Omega_Im_Minus) rotation_comp];
end


vel_Lines = [[Origin_Im Origin_Im Origin_Im Origin_Im];[Origin_Re Origin_Re Origin_Re Origin_Re];...
[Origin_Im Origin_Im+abs(Omega_Im_Minus) Origin_Im Origin_Im-abs(Omega_Im_Plus)];[Origin_Re+abs(Omega_Re_Plus) Origin_Re Origin_Re-abs(Omega_Re_Minus) Origin_Re]];

== matlab function Image Processing/Optical Flow/Cross for callibration/Optical Flow Lines1 ==
  data: vel_Values input double; Cam_Img_Dim input double; vel_Lines output double
function vel_Lines =OpticalFlowLines(vel_Values, Cam_Img_Dim) 

% Generates the coordinate points of optical flow lines

persistent first_time;
persistent X;
persistent Y;
persistent RV;
persistent CV;

%persistent Max_Vec_Length;

persistent Origin_Re;
persistent Origin_Im;

persistent Sec_1_Cnt;
persistent Sec_2_Cnt;
persistent Sec_3_Cnt;
persistent Sec_4_Cnt;

persistent Sec_1;
persistent Sec_2;
persistent Sec_3;
persistent Sec_4;

persistent R;
persistent C;
persistent Test_mat;
persistent med_vel_val;

%med_vel_val=median(vel_Values);
%[R C] = size(med_vel_val);
if isempty(first_time)
    first_time     = 1;
    Origin_Re = Cam_Img_Dim(1)/2%double(176);
    [R C] = size(vel_Values)
    Origin_Im = Cam_Img_Dim(2)/2%double(144);
end


Omega_Re_Plus = 700;
Omega_Re_Minus = 700;
Omega_Im_Plus = 700;
Omega_Im_Minus = 700;


vel_Lines = [[Origin_Im Origin_Im Origin_Im Origin_Im];[Origin_Re Origin_Re Origin_Re Origin_Re];...
[Origin_Im Origin_Im+abs(Omega_Im_Minus) Origin_Im Origin_Im-abs(Omega_Im_Plus)];[Origin_Re+abs(Omega_Re_Plus) Origin_Re Origin_Re-abs(Omega_Re_Minus) Origin_Re]];

== matlab function Image Processing/Optical Flow/Corner Features OF/Embedded MATLAB Function ==
  data: vec output double; Tform input double; allowNewCalc input double; rot output double; TsOpt input double
function [vec, rot] = clc(Tform, allowNewCalc, TsOpt)
%#eml
persistent vec_old;
persistent rot_old;
persistent first_time;
persistent db_3_filter;

if isempty(first_time)
    vec_old = double(complex(0,0));
    vec = double(complex(0,0));
    rot = double(0);
    rot_old = double(0);
    first_time=1;
    db_3_filter=double([0;0;0;0;0;0;0]);
end
    Tform
    %v'=Tform*v with v=[x y 1]^T and v'=[x' y' 1]
    if(allowNewCalc)
    vec=double(complex(Tform(2,3),Tform(1,3)));
    rot=double(abs(-asin(complex(Tform(1,2)))))/TsOpt;
    %Detect direction of rotation
    if((Tform(1,3) > 0) && Tform(2,3) < 0)
        %counterclockwise is negative
        rot=rot*(-1);
    end
    db_3_filter=circshift(db_3_filter, 1);
    db_3_filter(1,1)=rot;
    db_3_filter
    rot=sum(db_3_filter)/7;
    vec_old=vec;
    rot_old=rot;
else
vec=vec_old;
rot=rot_old;
end

== matlab function Image Processing/Optical Flow/Optical Flow Segmentation in Sectors Block Matching/Optical Flow Lines1 ==
  data: vel_Values input double; Cam_Img_Dim input double; vel_Lines output double; Omega_avg output double; scaleFactor parameter double size=1
function [vel_Lines, Omega_avg]=OpticalFlowLines(vel_Values, Cam_Img_Dim,scaleFactor) 

% Generates the coordinate points of optical flow lines

persistent first_time;
persistent X;
persistent Y;
persistent RV;
persistent CV;

%persistent Max_Vec_Length;

persistent Origin_Re;
persistent Origin_Im;

persistent Sec_1_Cnt;
persistent Sec_2_Cnt;
persistent Sec_3_Cnt;
persistent Sec_4_Cnt;

persistent Sec_1;
persistent Sec_2;
persistent Sec_3;
persistent Sec_4;

persistent R;
persistent C;
persistent Test_mat;
persistent med_vel_val;

%med_vel_val=median(vel_Values);
%[R C] = size(med_vel_val);
if isempty(first_time)
    first_time     = 1;
    Origin_Re = Cam_Img_Dim(1)/2%double(176);
    [R C] = size(vel_Values)
    Origin_Im = Cam_Img_Dim(2)/2%double(144);
end

Sec_1 = double(0);
Sec_2 = double(0);
Sec_3 = double(0);
Sec_4 = double(0);

Sec_1_Cnt = 1;
Sec_2_Cnt = 1;
Sec_3_Cnt = 1;
Sec_4_Cnt = 1;

%sectors
%       ^Im
%       |         
%   4   |  1
%-------------->Re
%   3   |  2
%       |

% for i=1:R
%     for k=1:C
%       j=vel_Values(i,k);
%     if(real(j)>=0) % Sec_1 or Sec_2
%         if(imag(j)>=0) %Sec_1
%             Sec_1_Cnt=Sec_1_Cnt+1;
%             Sec_1=Sec_1+double(abs(j))
%         else           %Sec_2
%             Sec_2_Cnt=Sec_2_Cnt+1;
%             Sec_2=Sec_2+double(abs(j))
%         end
%     else            % Sec_3 or Sec_4
%         if(imag(j)>=0) %Sec_4
%             Sec_4_Cnt=Sec_4_Cnt+1;
%             Sec_4=Sec_4+double(abs(j))
%         else           %Sec_3
%             Sec_3_Cnt=Sec_3_Cnt+1;
%             Sec_3=Sec_3+double(abs(j))
%         end
%     end
%     end
% end

%Other segm
for i=1:R
    for k=1:C
      j=vel_Values(i,k);
    if(real(j)>=0) % Sec_1 or Sec_2
        Sec_1_Cnt=Sec_1_Cnt+1;
        Sec_1=Sec_1+double(abs(real(j)));
        if(imag(j)>=0) %Sec_2
            Sec_2_Cnt=Sec_2_Cnt+1;
            Sec_2=Sec_2+double(imag(j));
        else           %Sec_4
            Sec_4_Cnt=Sec_4_Cnt+1;
            Sec_4=Sec_4+double(imag(j));
        end
    else            % Sec_3 or Sec_4
        Sec_3_Cnt=Sec_3_Cnt+1;
        Sec_3=Sec_3+double(abs(real(j)));
        if(imag(j)>=0) %Sec_2
            Sec_2_Cnt=Sec_2_Cnt+1;
            Sec_2=Sec_2+double(imag(j));
        else           %Sec_4
            Sec_4_Cnt=Sec_4_Cnt+1;
            Sec_4=Sec_4+double(imag(j));
        end
    end
    end
end


% Sec_1_Mat = vel_Values((real(vel_Values) >= 0) & (imag(vel_Values) >= 0));
% Sec_2_Mat = vel_Values((real(vel_Values) >= 0) & (imag(vel_Values) < 0));
% Sec_3_Mat = vel_Values((real(vel_Values) < 0) & (imag(vel_Values) < 0));
% Sec_4_Mat = vel_Values((real(vel_Values) < 0) & (imag(vel_Values) >= 0));


% Sec_1 = sum(abs(Sec_1_Mat)/(size(Sec_1_Mat, 1)*size(Sec_1_Mat, 2)));
% Sec_2 = sum(abs(Sec_1_Mat)/(size(Sec_1_Mat, 1)*size(Sec_1_Mat, 2)));
% Sec_3 = sum(abs(Sec_1_Mat)/(size(Sec_1_Mat, 1)*size(Sec_1_Mat, 2)));
% Sec_4 = sum(abs(Sec_1_Mat)/(size(Sec_1_Mat, 1)*size(Sec_1_Mat, 2)));

Sec_1 = Sec_1/Sec_1_Cnt;
Sec_2 = Sec_2/Sec_2_Cnt;
Sec_3 = Sec_3/Sec_3_Cnt;
Sec_4 = Sec_4/Sec_4_Cnt;

% Omega_Re_Plus = (scaleFactor*(Sec_1+Sec_2))/2
% Omega_Re_Minus = (scaleFactor*(Sec_3+Sec_4))/2
% Omega_Im_Plus = (scaleFactor*(Sec_1+Sec_4))/2
% Omega_Im_Minus = (scaleFactor*(Sec_3+Sec_2))/2

Omega_Re_Plus = scaleFactor*Sec_1; %Sec_2
Omega_Re_Minus = scaleFactor*Sec_3; %Sec_4
Omega_Im_Plus = scaleFactor*Sec_4; %Sec_1
Omega_Im_Minus = scaleFactor*Sec_2; %Sec_3

%Calculation of rotation

rotation_comp=min([abs(Omega_Re_Plus) abs(Omega_Re_Minus) abs(Omega_Im_Plus) abs(Omega_Im_Minus)]);

if(rotation_comp>0)
    Omega_avg = [abs(Omega_Re_Plus)-rotation_comp abs(Omega_Re_Minus)-rotation_comp abs(Omega_Im_Plus)-rotation_comp abs(Omega_Im_Minus)-rotation_comp rotation_comp];
else
    Omega_avg = [abs(Omega_Re_Plus) abs(Omega_Re_Minus) abs(Omega_Im_Plus) abs(Omega_Im_Minus) rotation_comp];
end


vel_Lines = [[Origin_Im Origin_Im Origin_Im Origin_Im];[Origin_Re Origin_Re Origin_Re Origin_Re];...
[Origin_Im Origin_Im+abs(Omega_Im_Minus) Origin_Im Origin_Im-abs(Omega_Im_Plus)];[Origin_Re+abs(Omega_Re_Plus) Origin_Re Origin_Re-abs(Omega_Re_Minus) Origin_Re]];

== matlab function Image Processing/Optical Flow/Optical Flow Lines1/Optical Flow Lines1 ==
  data: vel_Values input double; vel_Lines output double; dir_Vec output double; scaleFactor parameter double size=1
function [vel_Lines, dir_Vec]=OpticalFlowLines(vel_Values, scaleFactor) 

% Generates the coordinate points of optical flow lines

persistent first_time;
persistent X;
persistent Y;
persistent RV;
persistent CV;
if isempty(first_time)
    first_time     = 1;
    %% user may change the following three parameters
    borderOffset   = 5;
    decimFactorRow = 5;
    decimFactorCol = 5;    
    %%
    [R C] = size(vel_Values);
    RV = borderOffset:decimFactorRow:(R-borderOffset);   
    CV = borderOffset:decimFactorCol:(C-borderOffset);
    [Y X] = meshgrid(CV,RV);
end

tmp = vel_Values(RV,CV);
tmp = tmp.*(-1);
X(:)=180;Y(:)=180;
tmp=sum(tmp(:))/size(tmp(:), 2);
dir_Vec = scaleFactor*[real(tmp), imag(tmp)];
vel_Lines = [X(:)';Y(:)';X(:)'+imag(tmp(:))';Y(:)'+real(tmp(:))'];

== matlab function Image Processing/Optical Flow/Optical Flow Lines2/Optical Flow Lines1 ==
  data: vel_Values input double; vel_Lines output double; dir_Vec output double; scaleFactor parameter double size=1
function [vel_Lines, dir_Vec]=OpticalFlowLines(vel_Values, scaleFactor) 

% Generates the coordinate points of optical flow lines

persistent first_time;
persistent X;
persistent Y;
persistent RV;
persistent CV;
if isempty(first_time)
    first_time     = 1;
    %% user may change the following three parameters
    borderOffset   = 5;
    decimFactorRow = 5;
    decimFactorCol = 5;    
    %%
    [R C] = size(vel_Values);
    RV = borderOffset:decimFactorRow:(R-borderOffset);   
    CV = borderOffset:decimFactorCol:(C-borderOffset);
    [Y X] = meshgrid(CV,RV);
end

tmp = vel_Values(RV,CV);
tmp = tmp.*scaleFactor;
dir_Vec = scaleFactor*[real(tmp), imag(tmp)];
vel_Lines = [X(:)';Y(:)';X(:)'+imag(tmp(:))';Y(:)'+real(tmp(:))'];
